simulink model "HANcoder_E407_TTA_Controller_v2"  (R2018b)
settings: Solver=FixedStepDiscrete  StartTime=0.0  StopTime=1  FixedStep=0.01  RelTol=1e-3
PreLoadFcn:
  | librarySetup
  | eval([bdroot,'_startup']) %Calling [modelName]_startup.m
values from neighbouring files (symbols this model uses):
  basic_cycle_duration_bc0 = TM_Reset_Board   + COMP_duration    (= 212)    [HANcoder_E407_TTA_Controller_v3_startup.m]
  basic_cycle_duration_bc1 = TM_Reset_Var_bc1 + COMP_duration    (= 288)    [HANcoder_E407_TTA_Controller_v3_startup.m]
  comm_delay_estimation1 = round(comm_delay_measured1*hardware_granularity/frequency_IRQ)    [HANcoder_E407_TTA_Controller_v3_startup.m]
  comm_delay_estimation2 = round(comm_delay_measured2*hardware_granularity/frequency_IRQ)    [HANcoder_E407_TTA_Controller_v3_startup.m]
  COMM_Period = 40    [HANcoder_E407_TTA_Controller_v3_startup.m]
  COMM_Phase1 = Simulink.Parameter    [HANcoder_E407_TTA_Controller_v3_startup.m]
  COMM_Phase2 = Simulink.Parameter    [HANcoder_E407_TTA_Controller_v3_startup.m]
  COMP_duration = 4    [HANcoder_E407_TTA_Controller_v3_startup.m]
  Controller1_Board = 1    [HANcoder_E407_TTA_Controller_v3_startup.m]
  Controller2_Board = 2    [HANcoder_E407_TTA_Controller_v3_startup.m]
  Controller3_Board = 3    [HANcoder_E407_TTA_Controller_v3_startup.m]
  delta_max = 1    [HANcoder_E407_TTA_Controller_v3_startup.m]
  delta_min = -1    [HANcoder_E407_TTA_Controller_v3_startup.m]
  delta_precision = 6    [HANcoder_E407_TTA_Controller_v3_startup.m]
  e_width = 0.1    [HANcoder_E407_TTA_Controller_v3_startup.m]
  frequency_IRQ = 100    [HANcoder_E407_TTA_Controller_v3_startup.m]
  HANtuneOverride = Simulink.Parameter    [HANcoder_E407_TTA_Controller_v3_startup.m]
  hardware_granularity = 1000000    [HANcoder_E407_TTA_Controller_v3_startup.m]
  I_a = 2.25    [HANcoder_E407_TTA_Controller_v3_startup.m]
  I_f = 2.25    [HANcoder_E407_TTA_Controller_v3_startup.m]
  idle_time_init = basic_cycle_duration_bc0 + basic_cycle_duration_bc1    (= 500)    [HANcoder_E407_TTA_Controller_v3_startup.m]
  Input_Gen_Board = 4    [HANcoder_E407_TTA_Controller_v3_startup.m]
  LA_Clock_Gr = 1    [HANcoder_E407_TTA_Controller_v3_startup.m]
  LA_COMM_Err = 1    [HANcoder_E407_TTA_Controller_v3_startup.m]
  LA_MEX_Flag = 1    [HANcoder_E407_TTA_Controller_v3_startup.m]
  LA_Task_Act = 1    [HANcoder_E407_TTA_Controller_v3_startup.m]
  m_v = 100.0    (= 100)    [HANcoder_E407_TTA_Controller_v3_startup.m]
  Master_Role = 1    [HANcoder_E407_TTA_Controller_v3_startup.m]
  matrix_cycle_duration = basic_cycle_duration_bc0 + basic_cycle_duration_bc1    (= 500)    [HANcoder_E407_TTA_Controller_v3_startup.m]
  matrix_rows = 2    [HANcoder_E407_TTA_Controller_v3_startup.m]
  max_num_msgs_CAN1 = 2^Tx_bit_number-1    (= 7)    [HANcoder_E407_TTA_Controller_v3_startup.m]
  max_num_msgs_CAN2 = max_num_msgs_CAN1    (= 7)    [HANcoder_E407_TTA_Controller_v3_startup.m]
  OutControl1_ID = 23    [HANcoder_E407_TTA_Controller_v3_startup.m]
  OutControl2_ID = 24    [HANcoder_E407_TTA_Controller_v3_startup.m]
  OutEmulator_ID = 25    [HANcoder_E407_TTA_Controller_v3_startup.m]
  R_al = 0.10    (= 0.1)    [HANcoder_E407_TTA_Controller_v3_startup.m]
  R_ar = 0.10    (= 0.1)    [HANcoder_E407_TTA_Controller_v3_startup.m]
  R_fl = 0.10    (= 0.1)    [HANcoder_E407_TTA_Controller_v3_startup.m]
  R_fr = 0.10    (= 0.1)    [HANcoder_E407_TTA_Controller_v3_startup.m]
  SensorValues_ID = 22    [HANcoder_E407_TTA_Controller_v3_startup.m]
  SetValues_ID = 21    [HANcoder_E407_TTA_Controller_v3_startup.m]
  Slave_Role = 2    [HANcoder_E407_TTA_Controller_v3_startup.m]
  speed_k_d = Simulink.Parameter    [HANcoder_E407_TTA_Controller_v3_startup.m]
  speed_k_i = Simulink.Parameter    [HANcoder_E407_TTA_Controller_v3_startup.m]
  speed_k_p = Simulink.Parameter    [HANcoder_E407_TTA_Controller_v3_startup.m]
  speed_max = 10    [HANcoder_E407_TTA_Controller_v3_startup.m]
  speed_min = -10    [HANcoder_E407_TTA_Controller_v3_startup.m]
  speed_precision = 3    [HANcoder_E407_TTA_Controller_v3_startup.m]
  Sync_ID = 1    [HANcoder_E407_TTA_Controller_v3_startup.m]
  tau_max = 5    [HANcoder_E407_TTA_Controller_v3_startup.m]
  tau_min = -5    [HANcoder_E407_TTA_Controller_v3_startup.m]
  tau_range = abs(tau_max) + abs(tau_min)    [HANcoder_E407_TTA_Controller_v3_startup.m]
  theta_max = (speed_max/R_fr)*matrix_cycle_duration*frequency_IRQ/hardware_granularity    (= 5)    [HANcoder_E407_TTA_Controller_v3_startup.m]
  theta_min = (-1)*theta_max    (= -5)    [HANcoder_E407_TTA_Controller_v3_startup.m]
  theta_precision = 7-(fix(log2(theta_max))+1)    [HANcoder_E407_TTA_Controller_v3_startup.m]
  Tl_a = 0.6    [HANcoder_E407_TTA_Controller_v3_startup.m]
  Tl_f = 0.6    [HANcoder_E407_TTA_Controller_v3_startup.m]
  TM_Check_Output_Control1 = TM_COMM_Output_Control1 + COMM_duration    (= 188)    [HANcoder_E407_TTA_Controller_v3_startup.m]
  TM_Check_Output_Control2 = TM_COMM_Output_Control2 + COMM_duration    (= 232)    [HANcoder_E407_TTA_Controller_v3_startup.m]
  TM_Check_Output_Emulator = TM_COMM_Output_Emulator + COMM_duration    (= 280)    [HANcoder_E407_TTA_Controller_v3_startup.m]
  TM_Check_Sensor_Values = TM_COMM_Sensor_Values + COMM_duration    (= 132)    [HANcoder_E407_TTA_Controller_v3_startup.m]
  TM_Check_Set_Values = TM_COMM_Set_Values + COMM_duration    (= 88)    [HANcoder_E407_TTA_Controller_v3_startup.m]
  TM_Check_Sync = TM_COMM_Sync   + COMM_duration    (= 40)    [HANcoder_E407_TTA_Controller_v3_startup.m]
  TM_Check_TOuts = TM_Count_Vote3 + COMP_duration    (= 196)    [HANcoder_E407_TTA_Controller_v3_startup.m]
  TM_Check_Vote1 = TM_COMM_Vote1  + COMM_duration    (= 92)    [HANcoder_E407_TTA_Controller_v3_startup.m]
  TM_Check_Vote2 = TM_COMM_Vote2  + COMM_duration    (= 140)    [HANcoder_E407_TTA_Controller_v3_startup.m]
  TM_Check_Vote3 = TM_COMM_Vote3  + COMM_duration    (= 188)    [HANcoder_E407_TTA_Controller_v3_startup.m]
  TM_COMM_Output_Control1 = TM_Velocity + COMP_duration    (= 148)    [HANcoder_E407_TTA_Controller_v3_startup.m]
  TM_COMM_Output_Control2 = TM_Check_Output_Control1 + COMP_duration    (= 192)    [HANcoder_E407_TTA_Controller_v3_startup.m]
  TM_COMM_Output_Emulator = TM_TMR + COMP_duration    (= 240)    [HANcoder_E407_TTA_Controller_v3_startup.m]
  TM_COMM_Sensor_Values = TM_Check_Set_Values + COMP_duration    (= 92)    [HANcoder_E407_TTA_Controller_v3_startup.m]
  TM_COMM_Set_Values = TM_Update_LT + COMP_duration    (= 48)    [HANcoder_E407_TTA_Controller_v3_startup.m]
  TM_COMM_Sync = basic_cycle_start    (= 0)    [HANcoder_E407_TTA_Controller_v3_startup.m]
  TM_COMM_Vote1 = TM_Vote_Dec    + COMP_duration    (= 52)    [HANcoder_E407_TTA_Controller_v3_startup.m]
  TM_COMM_Vote2 = TM_Count_Vote1 + COMP_duration    (= 100)    [HANcoder_E407_TTA_Controller_v3_startup.m]
  TM_COMM_Vote3 = TM_Count_Vote2 + COMP_duration    (= 148)    [HANcoder_E407_TTA_Controller_v3_startup.m]
  TM_Count_Vote1 = TM_Check_Vote1 + COMP_duration    (= 96)    [HANcoder_E407_TTA_Controller_v3_startup.m]
  TM_Count_Vote2 = TM_Check_Vote2 + COMP_duration    (= 144)    [HANcoder_E407_TTA_Controller_v3_startup.m]
  TM_Count_Vote3 = TM_Check_Vote3 + COMP_duration    (= 192)    [HANcoder_E407_TTA_Controller_v3_startup.m]
  TM_Data_bc0 = TM_COMM_Sync    (= 0)    [HANcoder_E407_TTA_Controller_v3_startup.m]
  TM_Data_bc1 = TM_Data_bc0(1:4)    [HANcoder_E407_TTA_Controller_v3_startup.m]
  TM_New_Master = TM_Check_TOuts + COMP_duration    (= 200)    [HANcoder_E407_TTA_Controller_v3_startup.m]
  TM_Reset_Board = TM_Reset_Var   + COMP_duration    (= 208)    [HANcoder_E407_TTA_Controller_v3_startup.m]
  TM_Reset_Var = TM_New_Master  + COMP_duration    (= 204)    [HANcoder_E407_TTA_Controller_v3_startup.m]
  TM_Reset_Var_bc1 = TM_Check_Output_Emulator + COMP_duration    (= 284)    [HANcoder_E407_TTA_Controller_v3_startup.m]
  TM_Steer = TM_Check_Sensor_Values + COMP_duration    (= 136)    [HANcoder_E407_TTA_Controller_v3_startup.m]
  TM_TMR = TM_Check_Output_Control2 + COMP_duration    (= 236)    [HANcoder_E407_TTA_Controller_v3_startup.m]
  TM_Torque = TM_Steer + COMP_duration    (= 140)    [HANcoder_E407_TTA_Controller_v3_startup.m]
  TM_Type_bc0 = COMM    (= 0)    [HANcoder_E407_TTA_Controller_v3_startup.m]
  TM_Type_bc1 = TM_Type_bc0(1:4)    [HANcoder_E407_TTA_Controller_v3_startup.m]
  TM_Update_LT = TM_Check_Sync  + COMP_duration    (= 44)    [HANcoder_E407_TTA_Controller_v3_startup.m]
  TM_Velocity = TM_Torque + COMP_duration    (= 144)    [HANcoder_E407_TTA_Controller_v3_startup.m]
  TM_Vote_Dec = TM_Update_LT   + COMP_duration    (= 48)    [HANcoder_E407_TTA_Controller_v3_startup.m]
  torque_a_k_d = Simulink.Parameter    [HANcoder_E407_TTA_Controller_v3_startup.m]
  torque_a_k_i = Simulink.Parameter    [HANcoder_E407_TTA_Controller_v3_startup.m]
  torque_a_k_p = Simulink.Parameter    [HANcoder_E407_TTA_Controller_v3_startup.m]
  torque_f_k_d = Simulink.Parameter    [HANcoder_E407_TTA_Controller_v3_startup.m]
  torque_f_k_i = Simulink.Parameter    [HANcoder_E407_TTA_Controller_v3_startup.m]
  torque_f_k_p = Simulink.Parameter    [HANcoder_E407_TTA_Controller_v3_startup.m]
  torque_precision = 4    [HANcoder_E407_TTA_Controller_v3_startup.m]
  Vehicle_Em_Board = 5    [HANcoder_E407_TTA_Controller_v3_startup.m]
  Vote1_ID = 11    [HANcoder_E407_TTA_Controller_v3_startup.m]
  Vote2_ID = 12    [HANcoder_E407_TTA_Controller_v3_startup.m]
  Vote3_ID = 13    [HANcoder_E407_TTA_Controller_v3_startup.m]
undefined symbols (not defined in the file or in its folder): A0, A1, A2, A3, A4, CON2
libraries: hdlsllib x235, HANcoder_STM32_Target x25, simulink x3, simulink_extras x1
(part 5 of 22)

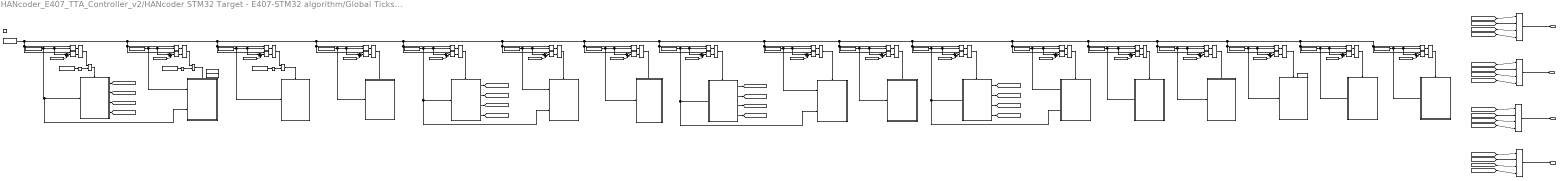
== system HANcoder_E407_TTA_Controller_v2/HANcoder STM32 Target - E407-STM32 algorithm/Global Ticks Increment/CAN Management/Matrix Cycle Manager/Subsystem/controller basic cycle 0 ==
  note: Output Send_Message
      | Send: 1
      | Do not send: 0
  note: Send message condition
      | Sync Msg: Master and TM0
      | Vote Msg: Node# and TM#
  note: Receive message condition
      | Sync Msg: Not Master and TM0
      | Vote Msg: Not # Node at TM#
  note: Receive message condition
      | Sync Msg: Not Master and TM0
      | Vote Msg: Not # Node at TM#
  note: Output Receive_Message
      | Receive: 1
      | Do not receive: 0
  note: Output Send_Message
      | Send: 1
      | Do not send: 0
  note: Output Receive_Message
      | Receive: 1
      | Do not receive: 0
  note: Send message condition
      | Sync Msg: Master and TM0
      | Vote Msg: Node# and TM#
  note: COMM - TW check
  note: COMP - TW check
  note: COMP - TW check
  note: COMP - TW check
  note: COMM - TW check
  note: COMP - TW check
  note: COMP - TW check
  note: COMM - TW check
  note: COMP - TW check
  note: COMP - TW check
  note: COMM - TW check
  note: COMP - TW check
  note: COMP - TW check
  note: COMP - TW check
  note: COMP - TW check
  note: COMP - TW check
  note: COMP - TW check
  note: Local Time still not updated
  note: Local Time still not updated
  note: Local Time still not updated
  Enable : EnablePort  PropagateVarSize=During execution
  AND{,1..19} (20 alike) : Logic  IconShape=distinctive  AllPortsSameDT=off  OutDataTypeStr=boolean
  COMM Task - Sync bc 0 : Subsystem
  COMM Task - Vote1 : Subsystem
  COMM Task - Vote2 : Subsystem
  COMM Task - Vote3 : Subsystem
  COMP Task - Check Timeouts : Subsystem
  COMP Task - New Master : Subsystem
  COMP Task - Reset Board : Subsystem
  COMP Task - Reset Variables BC0 : Subsystem
  COMP Task - Sync bc0 check : Subsystem
  COMP Task - Update LT : Subsystem
  COMP Task - Vote Decision : Subsystem
  COMP Task - Vote1 Count : Subsystem
  COMP Task - Vote1 check : Subsystem
  COMP Task - Vote2 Count : Subsystem
  COMP Task - Vote2 check : Subsystem
  COMP Task - Vote3 Count : Subsystem
  COMP Task - Vote3 check : Subsystem
  Constant : Constant  Value=TM_COMM_Sync
  Constant{1,4,10,29} (4 alike) : Constant  Value=COMM_Period
  Constant{5,7,11,13,15..16,18,20,22,24,26,30,32} (13 alike) : Constant  Value=COMP_duration
  Constant12 : Constant  Value=TM_Check_TOuts
  Constant14 : Constant  Value=TM_New_Master
  Constant17 : Constant  Value=TM_Update_LT
  Constant19 : Constant  Value=TM_Vote_Dec
  Constant2 : Constant  Value=TM_Check_Sync
  Constant21 : Constant  Value=TM_Count_Vote1
  Constant23 : Constant  Value=TM_Check_Vote3
  Constant25 : Constant  Value=TM_Reset_Var
  Constant27 : Constant  Value=TM_Count_Vote2
  Constant28 : Constant  Value=TM_COMM_Vote2
  Constant3 : Constant  Value=TM_COMM_Vote1
  Constant31 : Constant  Value=TM_Reset_Board
  Constant33 : Constant  Value=TM_Check_Vote2
  Constant6 : Constant  Value=TM_Check_Vote1
  Constant8 : Constant  Value=TM_Count_Vote3
  Constant9 : Constant  Value=TM_COMM_Vote3
  Data Store Memory11 : DataStoreMemory  DataStoreName=Msg_Rx  ReadBeforeWriteMsg=warning  WriteAfterWriteMsg=warning  WriteAfterReadMsg=warning  ShowAdditionalParam=off  OutDataTypeStr=Bus: msg_buffer_type
  Data Store Memory7 : DataStoreMemory  DataStoreName=Reset_Board  ReadBeforeWriteMsg=warning  WriteAfterWriteMsg=warning  WriteAfterReadMsg=warning  ShowAdditionalParam=off  OutDataTypeStr=boolean
  Data Store Memory8 : DataStoreMemory  DataStoreName=new_msg_Rx  ReadBeforeWriteMsg=warning  WriteAfterWriteMsg=warning  WriteAfterReadMsg=warning  ShowAdditionalParam=off
  Data Store Read11 : DataStoreRead  DataStoreName=BC0_Sync_processed
  Data Store Read6 : DataStoreRead  DataStoreName=BC0_Sync_processed
  Data Store Read7 : DataStoreRead  DataStoreName=BC0_Sync_processed
  Data Store Read8 : DataStoreRead  DataStoreName=Local_Ticks
  GreaterThan{,2,4,6,8,10,12,14,16,18,20,22,24,26,28,30,32} (17 alike) : RelationalOperator  OutDataTypeStr=boolean  RndMeth=Simplest
  GreaterThan{1,3,5,7,9,11,13,15,17,19,21,23,25,27,29,31,33} (17 alike) : RelationalOperator  Operator=<  OutDataTypeStr=boolean  RndMeth=Simplest
  NOT1 : Logic  Operator=NOT  IconShape=distinctive  AllPortsSameDT=off  OutDataTypeStr=boolean
  NOT2 : Logic  Operator=NOT  IconShape=distinctive  AllPortsSameDT=off  OutDataTypeStr=boolean
  NOT3 : Logic  Operator=NOT  IconShape=distinctive  AllPortsSameDT=off  OutDataTypeStr=boolean
  OR{1..4} (4 alike) : Logic  Operator=OR  Inputs=4  IconShape=distinctive  AllPortsSameDT=off  OutDataTypeStr=boolean
  Sum{1..17} (17 alike) : Sum  Inputs=|++
  Send_Message_CAN1 : Outport  OutputWhenDisabled=reset  InitialOutput=0
  Send_Message_CAN2 : Outport  Port=2  OutputWhenDisabled=reset  InitialOutput=0
  Receive_Message_CAN1 : Outport  Port=3  OutputWhenDisabled=reset  InitialOutput=0
  Receive_Message_CAN2 : Outport  Port=4  OutputWhenDisabled=reset  InitialOutput=0
  wires:
  OR1/1 -> Send_Message_CAN1/1
  [receive_CAN2_Sync_bc0_TAG] -> OR3/1
  [receive_CAN2_Vote3_bc0_TAG] -> OR3/4
  [receive_CAN2_Vote1_bc0_TAG] -> OR3/2
  [receive_CAN2_Vote2_bc0_TAG] -> OR3/3
  OR3/1 -> Receive_Message_CAN2/1
  [receive_CAN1_Sync_bc0_TAG] -> OR2/1
  [receive_CAN1_Vote1_bc0_TAG] -> OR2/2
  [receive_CAN1_Vote2_bc0_TAG] -> OR2/3
  [receive_CAN1_Vote3_bc0_TAG] -> OR2/4
  OR2/1 -> Receive_Message_CAN1/1
  [send_CAN2_Sync_bc0_TAG] -> OR4/1
  [send_CAN2_Vote1_bc0_TAG] -> OR4/2
  [send_CAN2_Vote2_bc0_TAG] -> OR4/3
  [send_CAN2_Vote3_bc0_TAG] -> OR4/4
  [send_CAN1_Sync_bc0_TAG] -> OR1/1
  [send_CAN1_Vote1_bc0_TAG] -> OR1/2
  [send_CAN1_Vote2_bc0_TAG] -> OR1/3
  [send_CAN1_Vote3_bc0_TAG] -> OR1/4
  OR4/1 -> Send_Message_CAN2/1
  COMM Task - Sync bc 0/1(Send CAN1) -> [send_CAN1_Sync_bc0_TAG]
  COMM Task - Sync bc 0/2(Receive CAN1) -> [receive_CAN1_Sync_bc0_TAG]
  COMM Task - Sync bc 0/3(Send CAN2) -> [send_CAN2_Sync_bc0_TAG]
  COMM Task - Sync bc 0/4(Receive CAN2) -> [receive_CAN2_Sync_bc0_TAG]
  Constant1/1 -> Sum4/2
  Constant/1 -> COMP Task - Sync bc0 check/2(TM_COMM), COMM Task - Sync bc 0/1(Time Mark), Sum4/1, GreaterThan/2
  Sum4/1 -> GreaterThan1/2
  GreaterThan/1 -> AND/1
  GreaterThan1/1 -> AND/2
  AND/1 -> AND17/1
  GreaterThan3/1 -> AND1/2
  GreaterThan2/1 -> AND1/1
  Sum1/1 -> GreaterThan3/2
  Constant2/1 -> COMP Task - Sync bc0 check/1(Time_Mark), GreaterThan2/2, Sum1/1
  Constant15/1 -> Sum1/2
  Constant16/1 -> Sum2/2
  Constant17/1 -> COMP Task - Update LT/1(Time_Mark), Sum2/1, GreaterThan4/2
  Sum2/1 -> GreaterThan5/2
  GreaterThan4/1 -> AND2/1
  GreaterThan5/1 -> AND2/2
  AND3/1 -> COMP Task - Vote Decision/Enable
  GreaterThan7/1 -> AND3/2
  GreaterThan6/1 -> AND3/1
  Sum3/1 -> GreaterThan7/2
  Constant19/1 -> COMP Task - Vote Decision/1(Time Mark), GreaterThan6/2, Sum3/1
  Constant18/1 -> Sum3/2
  COMM Task - Vote1/1(Send CAN1) -> [send_CAN1_Vote1_bc0_TAG]
  COMM Task - Vote1/2(Receive CAN1) -> [receive_CAN1_Vote1_bc0_TAG]
  COMM Task - Vote1/3(Send CAN2) -> [send_CAN2_Vote1_bc0_TAG]
  COMM Task - Vote1/4(Receive CAN2) -> [receive_CAN2_Vote1_bc0_TAG]
  GreaterThan9/1 -> AND4/2
  GreaterThan8/1 -> AND4/1
  Sum5/1 -> GreaterThan9/2
  Constant4/1 -> Sum5/2
  AND4/1 -> COMM Task - Vote1/Enable
  Constant3/1 -> COMP Task - Vote1 check/2(TM_COMM), COMM Task - Vote1/1(Time Mark), Sum5/1, GreaterThan8/2
  GreaterThan11/1 -> AND5/2
  Sum6/1 -> GreaterThan11/2
  GreaterThan10/1 -> AND5/1
  Constant5/1 -> Sum6/2
  Constant6/1 -> COMP Task - Vote1 check/1(Time_Mark), GreaterThan10/2, Sum6/1
  AND5/1 -> COMP Task - Vote1 check/Enable
  AND6/1 -> COMP Task - Vote1 Count/Enable
  Constant21/1 -> COMP Task - Vote1 Count/1(Time Mark), Sum7/1, GreaterThan12/2
  Constant20/1 -> Sum7/2
  GreaterThan12/1 -> AND6/1
  Sum7/1 -> GreaterThan13/2
  GreaterThan13/1 -> AND6/2
  GreaterThan17/1 -> AND9/2
  Sum10/1 -> GreaterThan17/2
  GreaterThan16/1 -> AND9/1
  Constant26/1 -> Sum10/2
  Constant27/1 -> COMP Task - Vote2 Count/1(Time Mark), GreaterThan16/2, Sum10/1
  AND9/1 -> COMP Task - Vote2 Count/Enable
  Constant33/1 -> COMP Task - Vote2 check/1(Time_Mark), Sum9/1, GreaterThan14/2
  Constant32/1 -> Sum9/2
  GreaterThan14/1 -> AND8/1
  Sum9/1 -> GreaterThan15/2
  GreaterThan15/1 -> AND8/2
  Constant28/1 -> COMP Task - Vote2 check/2(TM_COMM), COMM Task - Vote2/1(Time Mark), GreaterThan18/2, Sum8/1
  AND7/1 -> COMM Task - Vote2/Enable
  Constant29/1 -> Sum8/2
  Sum8/1 -> GreaterThan19/2
  GreaterThan18/1 -> AND7/1
  GreaterThan19/1 -> AND7/2
  COMM Task - Vote2/1(Send CAN1) -> [send_CAN1_Vote2_bc0_TAG]
  COMM Task - Vote2/2(Receive CAN1) -> [receive_CAN1_Vote2_bc0_TAG]
  COMM Task - Vote2/3(Send CAN2) -> [send_CAN2_Vote2_bc0_TAG]
  AND8/1 -> COMP Task - Vote2 check/Enable
  GreaterThan25/1 -> AND10/2
  GreaterThan24/1 -> AND10/1
  Sum12/1 -> GreaterThan25/2
  Constant10/1 -> Sum12/2
  Constant9/1 -> COMP Task - Vote3 check/2(TM_COMM), COMM Task - Vote3/1(Time Mark), Sum12/1, GreaterThan24/2
  GreaterThan21/1 -> AND11/2
  Sum13/1 -> GreaterThan21/2
  GreaterThan20/1 -> AND11/1
  Constant22/1 -> Sum13/2
  Constant23/1 -> COMP Task - Vote3 check/1(Time_Mark), GreaterThan20/2, Sum13/1
  AND12/1 -> COMP Task - Vote3 Count/Enable
  Constant8/1 -> COMP Task - Vote3 Count/1(Time Mark), Sum11/1, GreaterThan22/2
  Constant7/1 -> Sum11/2
  GreaterThan22/1 -> AND12/1
  Sum11/1 -> GreaterThan23/2
  GreaterThan23/1 -> AND12/2
  COMM Task - Vote3/1(Send CAN1) -> [send_CAN1_Vote3_bc0_TAG]
  COMM Task - Vote3/2(Receive CAN1) -> [receive_CAN1_Vote3_bc0_TAG]
  COMM Task - Vote3/3(Send CAN2) -> [send_CAN2_Vote3_bc0_TAG]
  COMM Task - Vote3/4(Receive CAN2) -> [receive_CAN2_Vote3_bc0_TAG]
  AND10/1 -> COMM Task - Vote3/Enable
  AND11/1 -> COMP Task - Vote3 check/Enable
  GreaterThan27/1 -> AND13/2
  Sum14/1 -> GreaterThan27/2
  GreaterThan26/1 -> AND13/1
  Constant11/1 -> Sum14/2
  Constant12/1 -> COMP Task - Check Timeouts/1(Time_Mark), GreaterThan26/2, Sum14/1
  AND13/1 -> COMP Task - Check Timeouts/Enable
  AND14/1 -> COMP Task - New Master/Enable
  Constant14/1 -> COMP Task - New Master/1(Time_Mark), Sum15/1, GreaterThan28/2
  Constant13/1 -> Sum15/2
  GreaterThan28/1 -> AND14/1
  Sum15/1 -> GreaterThan29/2
  GreaterThan29/1 -> AND14/2
  GreaterThan31/1 -> AND15/2
  Sum16/1 -> GreaterThan31/2
  GreaterThan30/1 -> AND15/1
  Constant24/1 -> Sum16/2
  Constant25/1 -> COMP Task - Reset Variables BC0/1(Time_Mark), GreaterThan30/2, Sum16/1
  AND15/1 -> COMP Task - Reset Variables BC0/Enable
  Data Store Read8/1 -> GreaterThan21/1, GreaterThan20/1, GreaterThan22/1, GreaterThan23/1, GreaterThan32/1, GreaterThan33/1, GreaterThan31/1, GreaterThan30/1, GreaterThan28/1, GreaterThan29/1, GreaterThan27/1, GreaterThan26/1, GreaterThan25/1, GreaterThan24/1, GreaterThan17/1, GreaterThan16/1, GreaterThan14/1, GreaterThan15/1, GreaterThan18/1, GreaterThan19/1, GreaterThan12/1, GreaterThan13/1, GreaterThan11/1, GreaterThan10/1, GreaterThan9/1, GreaterThan8/1, GreaterThan6/1, GreaterThan7/1, GreaterThan4/1, GreaterThan5/1, GreaterThan2/1, GreaterThan3/1, GreaterThan/1, GreaterThan1/1
  AND16/1 -> COMP Task - Reset Board/Enable
  Constant31/1 -> COMP Task - Reset Board/1(Time_Mark), Sum17/1, GreaterThan32/2
  Constant30/1 -> Sum17/2
  GreaterThan32/1 -> AND16/1
  Sum17/1 -> GreaterThan33/2
  GreaterThan33/1 -> AND16/2
  Data Store Read11/1 -> NOT2/1
  NOT2/1 -> AND17/2
  AND17/1 -> COMM Task - Sync bc 0/Enable
  Data Store Read6/1 -> NOT1/1
  NOT1/1 -> AND18/2
  AND1/1 -> AND18/1
  AND18/1 -> COMP Task - Sync bc0 check/Enable
  Data Store Read7/1 -> NOT3/1
  NOT3/1 -> AND19/2
  AND2/1 -> AND19/1
  AND19/1 -> COMP Task - Update LT/Enable
  COMM Task - Vote2/4(Receive CAN2) -> [receive_CAN2_Vote2_bc0_TAG]

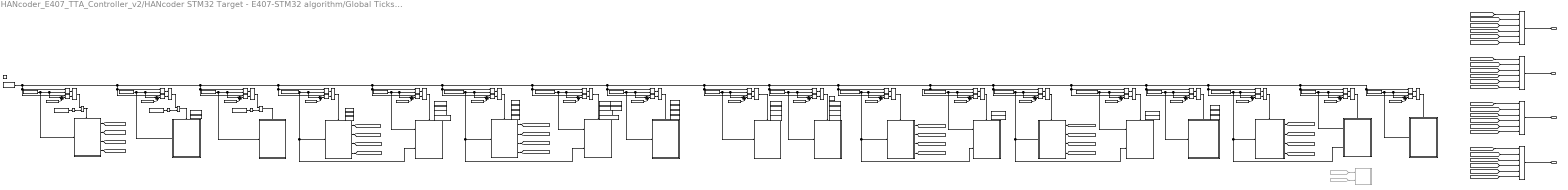
== system HANcoder_E407_TTA_Controller_v2/HANcoder STM32 Target - E407-STM32 algorithm/Global Ticks Increment/CAN Management/Matrix Cycle Manager/Subsystem/controller basic cycle 1 ==
  note: Receive message condition
      | Sync Msg: Not Master and TM0
      | Vote Msg: Not # Node at TM#
  note: Send message condition
      | Sync Msg: Master and TM0
      | Vote Msg: Node# and TM#
  note: Output Send_Message
      | Send: 1
      | Do not send: 0
  note: Output Receive_Message
      | Receive: 1
      | Do not receive: 0
  note: Output Receive_Message
      | Receive: 1
      | Do not receive: 0
  note: Output Send_Message
      | Send: 1
      | Do not send: 0
  note: Send message condition
      | Sync Msg: Master and TM0
      | Vote Msg: Node# and TM#
  note: Receive message condition
      | Sync Msg: Not Master and TM0
      | Vote Msg: Not # Node at TM#
  note: COMM - TW check
  note: COMP - TW check
  note: COMM - TW check
  note: COMP - TW check
  note: COMP - TW check
  note: COMP - TW check
  note: COMP - TW check
  note: COMM - TW check
  note: COMP - TW check
  note: COMP - TW check
  note: COMP - TW check
  note: Local Time still not updated
  note: COMP - TW check
  note: COMP - TW check
  note: Local Time still not updated
  note: COMP - TW check
  note: COMP - TW check
  note: COMM - TW check
  note: Local Time still not updated
  note: COMM - TW check
  note: COMP - TW check
  Enable : EnablePort
  AND{,1..20} (21 alike) : Logic  IconShape=distinctive  AllPortsSameDT=off  OutDataTypeStr=boolean
  COMM Task - Output Control1 : Subsystem
  COMM Task - Output Control2 : Subsystem
  COMM Task - Output Emulator : Subsystem
  COMM Task - Sensor_Values : Subsystem
  COMM Task - Set_Values : Subsystem
  COMM Task - Sync bc 1 : Subsystem
  COMP Task - Calculate Speed : Subsystem
  COMP Task - Calculate Steer : Subsystem
  COMP Task - Calculate Torque : Subsystem
  COMP Task - Estimate Vehicle States : Subsystem  Commented=on
  COMP Task - Reset Variables BC1 : Subsystem
  COMP Task - Rx_Output_Control1_Check : Subsystem
  COMP Task - Rx_Output_Control2_Check : Subsystem
  COMP Task - Rx_Output_Emulator_Check : Subsystem
  COMP Task - Rx_Sensor_Values_Check : Subsystem
  COMP Task - Rx_Set_Values_Check : Subsystem
  COMP Task - Sync bc1 check : Subsystem
  COMP Task - TMR : Subsystem
  COMP Task - Update LT : Subsystem
  Constant : Constant  Value=TM_COMM_Sync
  Constant{1,10,18,24,34,36} (6 alike) : Constant  Value=COMM_Period
  Constant{2..3,8..9,11,13,15,20,22,26,29..30} (12 alike) : Constant  Value=COMP_duration
  Constant12 : Constant  Value=TM_Check_Output_Control2
  Constant14 : Constant  Value=TM_TMR
  Constant16 : Constant  Value=TM_Reset_Var_bc1
  Constant21 : Constant  Value=TM_Check_Sensor_Values
  Constant23 : Constant  Value=TM_Check_Output_Control1
  Constant25 : Constant  Value=TM_COMM_Output_Emulator
  Constant27 : Constant  Value=TM_Velocity
  Constant28 : Constant  Value=TM_Steer
  Constant31 : Constant  Value=TM_Reset_Board
  Constant33 : Constant  Value=TM_Torque
  Constant35 : Constant  Value=TM_COMM_Sensor_Values
  Constant37 : Constant  Value=TM_COMM_Output_Control2
  Constant38 : Constant  Value=TM_COMM_Output_Control1
  Constant4 : Constant  Value=TM_Update_LT
  Constant5 : Constant  Value=TM_COMM_Set_Values
  Constant6 : Constant  Value=TM_Check_Sync
  Constant7 : Constant  Value=TM_Check_Set_Values
  Data Store Memory10 : DataStoreMemory  DataStoreName=v_set_stored  ReadBeforeWriteMsg=warning  WriteAfterWriteMsg=warning  WriteAfterReadMsg=warning  ShowAdditionalParam=off
  Data Store Memory11 : DataStoreMemory  DataStoreName=Msg_Rx  ReadBeforeWriteMsg=warning  WriteAfterWriteMsg=warning  WriteAfterReadMsg=warning  ShowAdditionalParam=off  OutDataTypeStr=Bus: msg_buffer_type
  Data Store Memory13 : DataStoreMemory  DataStoreName=theta_ar_stored  ReadBeforeWriteMsg=warning  WriteAfterWriteMsg=warning  WriteAfterReadMsg=warning  ShowAdditionalParam=off
  Data Store Memory14 : DataStoreMemory  DataStoreName=theta_al_stored  ReadBeforeWriteMsg=warning  WriteAfterWriteMsg=warning  WriteAfterReadMsg=warning  ShowAdditionalParam=off
  Data Store Memory18 : DataStoreMemory  DataStoreName=rx_data_incr_time  ReadBeforeWriteMsg=warning  WriteAfterWriteMsg=warning  WriteAfterReadMsg=warning  InitialValue=1  ShowAdditionalParam=off
  Data Store Memory19 : DataStoreMemory  DataStoreName=output_control1_rx  ReadBeforeWriteMsg=warning  WriteAfterWriteMsg=warning  WriteAfterReadMsg=warning  ShowAdditionalParam=off
  Data Store Memory20 : DataStoreMemory  DataStoreName=delta_f_set_stored  ReadBeforeWriteMsg=warning  WriteAfterWriteMsg=warning  WriteAfterReadMsg=warning  ShowAdditionalParam=off
  Data Store Memory21 : DataStoreMemory  DataStoreName=torque_fr_out  ReadBeforeWriteMsg=warning  WriteAfterWriteMsg=warning  WriteAfterReadMsg=warning  ShowAdditionalParam=off
  Data Store Memory22 : DataStoreMemory  DataStoreName=torque_fl_out  ReadBeforeWriteMsg=warning  WriteAfterWriteMsg=warning  WriteAfterReadMsg=warning  ShowAdditionalParam=off
  Data Store Memory23 : DataStoreMemory  DataStoreName=v_set  ReadBeforeWriteMsg=warning  WriteAfterWriteMsg=warning  WriteAfterReadMsg=warning  ShowAdditionalParam=off
  Data Store Memory24 : DataStoreMemory  DataStoreName=delta_f_set  ReadBeforeWriteMsg=warning  WriteAfterWriteMsg=warning  WriteAfterReadMsg=warning  ShowAdditionalParam=off
  Data Store Memory25 : DataStoreMemory  DataStoreName=torque_ar_out  ReadBeforeWriteMsg=warning  WriteAfterWriteMsg=warning  WriteAfterReadMsg=warning  ShowAdditionalParam=off
  Data Store Memory26 : DataStoreMemory  DataStoreName=torque_al_out  ReadBeforeWriteMsg=warning  WriteAfterWriteMsg=warning  WriteAfterReadMsg=warning  ShowAdditionalParam=off
  Data Store Memory27 : DataStoreMemory  DataStoreName=delta_a_set  ReadBeforeWriteMsg=warning  WriteAfterWriteMsg=warning  WriteAfterReadMsg=warning  ShowAdditionalParam=off
  Data Store Memory28 : DataStoreMemory  DataStoreName=Error_SetValues_NotRX  ReadBeforeWriteMsg=warning  WriteAfterWriteMsg=warning  WriteAfterReadMsg=warning  ShowAdditionalParam=off  OutDataTypeStr=boolean
  Data Store Memory30 : DataStoreMemory  DataStoreName=Error_SensorValues_NotRX  ReadBeforeWriteMsg=warning  WriteAfterWriteMsg=warning  WriteAfterReadMsg=warning  ShowAdditionalParam=off  OutDataTypeStr=boolean
  Data Store Memory31 : DataStoreMemory  DataStoreName=delta_a_set_stored  ReadBeforeWriteMsg=warning  WriteAfterWriteMsg=warning  WriteAfterReadMsg=warning  ShowAdditionalParam=off
  Data Store Memory33 : DataStoreMemory  DataStoreName=theta_fr  ReadBeforeWriteMsg=warning  WriteAfterWriteMsg=warning  WriteAfterReadMsg=warning  ShowAdditionalParam=off
  Data Store Memory34 : DataStoreMemory  DataStoreName=theta_dot_fr  ReadBeforeWriteMsg=warning  WriteAfterWriteMsg=warning  WriteAfterReadMsg=warning  ShowAdditionalParam=off
  Data Store Memory35 : DataStoreMemory  DataStoreName=theta_dot_ar  ReadBeforeWriteMsg=warning  WriteAfterWriteMsg=warning  WriteAfterReadMsg=warning  ShowAdditionalParam=off
  Data Store Memory36 : DataStoreMemory  DataStoreName=theta_dot_fl  ReadBeforeWriteMsg=warning  WriteAfterWriteMsg=warning  WriteAfterReadMsg=warning  ShowAdditionalParam=off
  Data Store Memory37 : DataStoreMemory  DataStoreName=theta_dot_al  ReadBeforeWriteMsg=warning  WriteAfterWriteMsg=warning  WriteAfterReadMsg=warning  ShowAdditionalParam=off
  Data Store Memory38 : DataStoreMemory  DataStoreName=v_est  ReadBeforeWriteMsg=warning  WriteAfterWriteMsg=warning  WriteAfterReadMsg=warning  ShowAdditionalParam=off
  Data Store Memory39 : DataStoreMemory  DataStoreName=torque_fr_set  ReadBeforeWriteMsg=warning  WriteAfterWriteMsg=warning  WriteAfterReadMsg=warning  ShowAdditionalParam=off
  Data Store Memory40 : DataStoreMemory  DataStoreName=torque_fl_set  ReadBeforeWriteMsg=warning  WriteAfterWriteMsg=warning  WriteAfterReadMsg=warning  ShowAdditionalParam=off
  Data Store Memory41 : DataStoreMemory  DataStoreName=torque_ar_set  ReadBeforeWriteMsg=warning  WriteAfterWriteMsg=warning  WriteAfterReadMsg=warning  ShowAdditionalParam=off
  Data Store Memory42 : DataStoreMemory  DataStoreName=torque_al_set  ReadBeforeWriteMsg=warning  WriteAfterWriteMsg=warning  WriteAfterReadMsg=warning  ShowAdditionalParam=off
  Data Store Memory43 : DataStoreMemory  DataStoreName=theta_fl  ReadBeforeWriteMsg=warning  WriteAfterWriteMsg=warning  WriteAfterReadMsg=warning  ShowAdditionalParam=off
  Data Store Memory44 : DataStoreMemory  DataStoreName=theta_ar  ReadBeforeWriteMsg=warning  WriteAfterWriteMsg=warning  WriteAfterReadMsg=warning  ShowAdditionalParam=off
  Data Store Memory46 : DataStoreMemory  DataStoreName=theta_al  ReadBeforeWriteMsg=warning  WriteAfterWriteMsg=warning  WriteAfterReadMsg=warning  ShowAdditionalParam=off
  Data Store Memory47 : DataStoreMemory  DataStoreName=output_control1_msg  ReadBeforeWriteMsg=warning  WriteAfterWriteMsg=warning  WriteAfterReadMsg=warning  ShowAdditionalParam=off  OutDataTypeStr=Bus: msg_buffer_type
  Data Store Memory48 : DataStoreMemory  DataStoreName=output_control2_rx  ReadBeforeWriteMsg=warning  WriteAfterWriteMsg=warning  WriteAfterReadMsg=warning  ShowAdditionalParam=off
  Data Store Memory49 : DataStoreMemory  DataStoreName=output_control2_msg  ReadBeforeWriteMsg=warning  WriteAfterWriteMsg=warning  WriteAfterReadMsg=warning  ShowAdditionalParam=off  OutDataTypeStr=Bus: msg_buffer_type
  Data Store Memory50 : DataStoreMemory  DataStoreName=error_log_1  ReadBeforeWriteMsg=warning  WriteAfterWriteMsg=warning  WriteAfterReadMsg=warning  ShowAdditionalParam=off  OutDataTypeStr=uint8
  Data Store Memory51 : DataStoreMemory  DataStoreName=theta_fr_stored  ReadBeforeWriteMsg=warning  WriteAfterWriteMsg=warning  WriteAfterReadMsg=warning  ShowAdditionalParam=off
  Data Store Memory52 : DataStoreMemory  DataStoreName=theta_fl_stored  ReadBeforeWriteMsg=warning  WriteAfterWriteMsg=warning  WriteAfterReadMsg=warning  ShowAdditionalParam=off
  Data Store Memory53 : DataStoreMemory  DataStoreName=error_log_2  ReadBeforeWriteMsg=warning  WriteAfterWriteMsg=warning  WriteAfterReadMsg=warning  ShowAdditionalParam=off  OutDataTypeStr=uint8
  Data Store Memory54 : DataStoreMemory  DataStoreName=error_log_3  ReadBeforeWriteMsg=warning  WriteAfterWriteMsg=warning  WriteAfterReadMsg=warning  ShowAdditionalParam=off  OutDataTypeStr=uint8
  Data Store Memory8 : DataStoreMemory  DataStoreName=new_msg_Rx  ReadBeforeWriteMsg=warning  WriteAfterWriteMsg=warning  WriteAfterReadMsg=warning  ShowAdditionalParam=off
  Data Store Read1 : DataStoreRead  DataStoreName=Local_Ticks
  Data Store Read11 : DataStoreRead  DataStoreName=BC1_Sync_processed
  Data Store Read6 : DataStoreRead  DataStoreName=BC1_Sync_processed
  Data Store Read7 : DataStoreRead  DataStoreName=BC1_Sync_processed
  From180 : From  Commented=on  GotoTag=basic_cycle_TAG
  From181 : From  Commented=on  GotoTag=local_ticks_TAG
  GreaterThan{,2,4,6,8,10,12,14,16,18,20,22,24,26,28,30,32,34} (18 alike) : RelationalOperator  OutDataTypeStr=boolean  RndMeth=Simplest
  GreaterThan{1,3,5,7,9,11,13,15,17,19,21,23,25,27,29,31,33,35} (18 alike) : RelationalOperator  Operator=<  OutDataTypeStr=boolean  RndMeth=Simplest
  NOT2 : Logic  Operator=NOT  IconShape=distinctive  AllPortsSameDT=off  OutDataTypeStr=boolean
  NOT4 : Logic  Operator=NOT  IconShape=distinctive  AllPortsSameDT=off  OutDataTypeStr=boolean
  NOT5 : Logic  Operator=NOT  IconShape=distinctive  AllPortsSameDT=off  OutDataTypeStr=boolean
  OR{1..4} (4 alike) : Logic  Operator=OR  Inputs=6  IconShape=distinctive  AllPortsSameDT=off  OutDataTypeStr=boolean
  Sum{1..18} (18 alike) : Sum  Inputs=|++
  Send_Message_CAN1 : Outport  OutputWhenDisabled=reset  InitialOutput=0
  Send_Message_CAN2 : Outport  Port=2  OutputWhenDisabled=reset  InitialOutput=0
  Receive_Message_CAN1 : Outport  Port=3  OutputWhenDisabled=reset  InitialOutput=0
  Receive_Message_CAN2 : Outport  Port=4  OutputWhenDisabled=reset  InitialOutput=0
  wires:
  COMM Task - Sensor_Values/3(Send CAN2) -> [send_CAN2_Sensor_Values_bc1_TAG]
  COMM Task - Sensor_Values/1(Send CAN1) -> [send_CAN1_Sensor_Values_bc1_TAG]
  COMM Task - Sensor_Values/2(Receive CAN1) -> [receive_CAN1_Sensor_Values_bc1_TAG]
  COMM Task - Sensor_Values/4(Receive CAN2) -> [receive_CAN2_Sensor_Values_bc1_TAG]
  From181/1 -> COMP Task - Estimate Vehicle States/2(local time)
  From180/1 -> COMP Task - Estimate Vehicle States/1(basic cycle)
  OR1/1 -> Send_Message_CAN1/1
  OR2/1 -> Receive_Message_CAN2/1
  OR4/1 -> Send_Message_CAN2/1
  OR3/1 -> Receive_Message_CAN1/1
  [send_CAN1_Sync_bc1_TAG] -> OR1/1
  [send_CAN1_Set_Values_bc1_TAG] -> OR1/2
  [send_CAN1_Sensor_Values_bc1_TAG] -> OR1/3
  [send_CAN1_Out_Control1_bc1_TAG] -> OR1/4
  [send_CAN1_Out_Control2_bc1_TAG] -> OR1/5
  [send_CAN1_Out_Emulator_bc1_TAG] -> OR1/6
  [send_CAN2_Sync_bc1_TAG] -> OR4/1
  [send_CAN2_Set_Values_bc1_TAG] -> OR4/2
  [send_CAN2_Sensor_Values_bc1_TAG] -> OR4/3
  [send_CAN2_Out_Control1_bc1_TAG] -> OR4/4
  [send_CAN2_Out_Control2_bc1_TAG] -> OR4/5
  [send_CAN2_Out_Emulator_bc1_TAG] -> OR4/6
  [receive_CAN1_Sync_bc1_TAG] -> OR3/1
  [receive_CAN1_Set_Values_bc1_TAG] -> OR3/2
  [receive_CAN1_Sensor_Values_bc1_TAG] -> OR3/3
  [receive_CAN1_Out_Control1_bc1_TAG] -> OR3/4
  [receive_CAN1_Out_Emulator_bc1_TAG] -> OR3/6
  [receive_CAN1_Out_Control2_bc1_TAG] -> OR3/5
  [receive_CAN2_Sync_bc1_TAG] -> OR2/1
  [receive_CAN2_Set_Values_bc1_TAG] -> OR2/2
  [receive_CAN2_Out_Control1_bc1_TAG] -> OR2/4
  [receive_CAN2_Sensor_Values_bc1_TAG] -> OR2/3
  [receive_CAN2_Out_Control2_bc1_TAG] -> OR2/5
  [receive_CAN2_Out_Emulator_bc1_TAG] -> OR2/6
  AND11/1 -> COMP Task - Rx_Output_Control1_Check/Enable
  AND12/1 -> COMM Task - Output Control2/Enable
  Constant1/1 -> Sum4/2
  COMM Task - Sync bc 1/1(Send CAN1) -> [send_CAN1_Sync_bc1_TAG]
  COMM Task - Sync bc 1/2(Receive CAN1) -> [receive_CAN1_Sync_bc1_TAG]
  COMM Task - Sync bc 1/4(Receive CAN2) -> [receive_CAN2_Sync_bc1_TAG]
  GreaterThan18/1 -> AND7/1
  AND19/1 -> COMP Task - Update LT/Enable
  AND4/1 -> COMP Task - Rx_Set_Values_Check/Enable
  Constant38/1 -> COMP Task - Rx_Output_Control1_Check/2(TM_COMM), COMM Task - Output Control1/1(Time Mark), Sum12/1, GreaterThan24/2
  GreaterThan29/1 -> AND14/2
  NOT2/1 -> AND18/2
  Constant14/1 -> COMP Task - TMR/1(Time_Mark), Sum15/1, GreaterThan28/2
  Sum15/1 -> GreaterThan29/2
  GreaterThan24/1 -> AND10/1
  GreaterThan16/1 -> AND9/1
  Constant9/1 -> Sum5/2
  GreaterThan22/1 -> AND12/1
  Sum14/1 -> GreaterThan27/2
  Data Store Read7/1 -> NOT5/1
  GreaterThan4/1 -> AND2/1
  Constant31/1 -> COMP Task - Rx_Output_Emulator_Check/1(Time_Mark), Sum17/1, GreaterThan32/2
  AND3/1 -> COMM Task - Set_Values/Enable
  GreaterThan28/1 -> AND14/1
  AND18/1 -> COMP Task - Sync bc1 check/Enable
  GreaterThan12/1 -> AND6/1
  AND1/1 -> AND18/1
  Sum17/1 -> GreaterThan33/2
  Constant30/1 -> Sum17/2
  GreaterThan20/1 -> AND11/1
  Data Store Read11/1 -> NOT4/1
  AND13/1 -> COMP Task - Rx_Output_Control2_Check/Enable
  AND17/1 -> COMM Task - Sync bc 1/Enable
  GreaterThan25/1 -> AND10/2
  GreaterThan33/1 -> AND16/2
  AND2/1 -> AND19/1
  GreaterThan32/1 -> AND16/1
  Data Store Read6/1 -> NOT2/1
  NOT4/1 -> AND17/2
  GreaterThan23/1 -> AND12/2
  AND15/1 -> COMM Task - Output Emulator/Enable
  AND14/1 -> COMP Task - TMR/Enable
  AND16/1 -> COMP Task - Rx_Output_Emulator_Check/Enable
  GreaterThan30/1 -> AND15/1
  Sum16/1 -> GreaterThan31/2
  Constant24/1 -> Sum16/2
  Constant25/1 -> COMP Task - Rx_Output_Emulator_Check/2(TM_COMM), COMM Task - Output Emulator/1(Time Mark), GreaterThan30/2, Sum16/1
  Constant27/1 -> COMP Task - Calculate Speed/1(Time_Mark), GreaterThan16/2, Sum10/1
  GreaterThan21/1 -> AND11/2
  GreaterThan1/1 -> AND/2
  Constant13/1 -> Sum15/2
  GreaterThan/1 -> AND/1
  Constant37/1 -> Sum11/1, GreaterThan22/2, COMP Task - Rx_Output_Control2_Check/2(TM_COMM), COMM Task - Output Control2/1(Time Mark)
  Constant20/1 -> Sum7/2
  Constant12/1 -> COMP Task - Rx_Output_Control2_Check/1(Time_Mark), GreaterThan26/2, Sum14/1
  GreaterThan10/1 -> AND5/1
  Constant/1 -> COMM Task - Sync bc 1/1(Time Mark), Sum4/1, GreaterThan/2
  GreaterThan26/1 -> AND13/1
  Constant11/1 -> Sum14/2
  AND7/1 -> COMP Task - Calculate Steer/Enable
  Constant23/1 -> COMP Task - Rx_Output_Control1_Check/1(Time_Mark), GreaterThan20/2, Sum13/1
  Constant5/1 -> COMM Task - Set_Values/1(Time Mark), COMP Task - Rx_Set_Values_Check/2(TM_COMM), GreaterThan6/2, Sum3/1
  Sum12/1 -> GreaterThan25/2
  Sum11/1 -> GreaterThan23/2
  Constant18/1 -> Sum3/2
  Constant22/1 -> Sum13/2
  GreaterThan19/1 -> AND7/2
  Sum8/1 -> GreaterThan19/2
  Constant10/1 -> Sum12/2
  Sum9/1 -> GreaterThan15/2
  Constant29/1 -> Sum8/2
  AND/1 -> AND17/1
  Constant28/1 -> COMP Task - Calculate Steer/1(Time_Mark), GreaterThan18/2, Sum8/1
  GreaterThan15/1 -> AND8/2
  Constant26/1 -> Sum10/2
  Sum10/1 -> GreaterThan17/2
  GreaterThan14/1 -> AND8/1
  Constant8/1 -> Sum9/2
  Sum7/1 -> GreaterThan13/2
  Constant36/1 -> Sum11/2
  Sum6/1 -> GreaterThan11/2
  Constant3/1 -> Sum2/2
  Constant35/1 -> COMP Task - Rx_Sensor_Values_Check/2(TM_COMM), COMM Task - Sensor_Values/1(Time Mark), GreaterThan10/2, Sum6/1
  Constant7/1 -> COMP Task - Rx_Set_Values_Check/1(Time_Mark), Sum5/1, GreaterThan8/2
  GreaterThan17/1 -> AND9/2
  AND10/1 -> COMM Task - Output Control1/Enable
  Sum3/1 -> GreaterThan7/2
  Constant4/1 -> COMP Task - Update LT/1(Time_Mark), Sum2/1, GreaterThan4/2
  Sum5/1 -> GreaterThan9/2
  Sum4/1 -> GreaterThan1/2
  AND5/1 -> COMM Task - Sensor_Values/Enable
  GreaterThan6/1 -> AND3/1
  GreaterThan8/1 -> AND4/1
  GreaterThan9/1 -> AND4/2
  GreaterThan31/1 -> AND15/2
  AND8/1 -> COMP Task - Calculate Torque/Enable
  GreaterThan13/1 -> AND6/2
  Sum13/1 -> GreaterThan21/2
  GreaterThan2/1 -> AND1/1
  GreaterThan3/1 -> AND1/2
  Constant2/1 -> Sum1/2
  GreaterThan7/1 -> AND3/2
  Constant6/1 -> COMP Task - Sync bc1 check/1(Time_Mark), GreaterThan2/2, Sum1/1
  AND6/1 -> COMP Task - Rx_Sensor_Values_Check/Enable
  GreaterThan11/1 -> AND5/2
  Sum1/1 -> GreaterThan3/2
  Constant34/1 -> Sum6/2
  AND9/1 -> COMP Task - Calculate Speed/Enable
  COMM Task - Sync bc 1/3(Send CAN2) -> [send_CAN2_Sync_bc1_TAG]
  Constant33/1 -> COMP Task - Calculate Torque/1(Time_Mark), Sum9/1, GreaterThan14/2
  GreaterThan27/1 -> AND13/2
  Constant21/1 -> COMP Task - Rx_Sensor_Values_Check/1(Time_Mark), Sum7/1, GreaterThan12/2
  NOT5/1 -> AND19/2
  Sum2/1 -> GreaterThan5/2
  GreaterThan5/1 -> AND2/2
  COMM Task - Set_Values/1(Send CAN1) -> [send_CAN1_Set_Values_bc1_TAG]
  COMM Task - Set_Values/2(Receive CAN1) -> [receive_CAN1_Set_Values_bc1_TAG]
  COMM Task - Set_Values/3(Send CAN2) -> [send_CAN2_Set_Values_bc1_TAG]
  COMM Task - Set_Values/4(Receive CAN2) -> [receive_CAN2_Set_Values_bc1_TAG]
  COMM Task - Output Control1/1(Send CAN1) -> [send_CAN1_Out_Control1_bc1_TAG]
  COMM Task - Output Control1/2(Receive CAN1) -> [receive_CAN1_Out_Control1_bc1_TAG]
  COMM Task - Output Control1/4(Receive CAN2) -> [receive_CAN2_Out_Control1_bc1_TAG]
  COMM Task - Output Control1/3(Send CAN2) -> [send_CAN2_Out_Control1_bc1_TAG]
  COMM Task - Output Control2/1(Send CAN1) -> [send_CAN1_Out_Control2_bc1_TAG]
  COMM Task - Output Control2/2(Receive CAN1) -> [receive_CAN1_Out_Control2_bc1_TAG]
  COMM Task - Output Control2/3(Send CAN2) -> [send_CAN2_Out_Control2_bc1_TAG]
  COMM Task - Output Control2/4(Receive CAN2) -> [receive_CAN2_Out_Control2_bc1_TAG]
  GreaterThan35/1 -> AND20/2
  Constant16/1 -> Sum18/1, GreaterThan34/2, COMP Task - Reset Variables BC1/1(Time_Mark)
  Constant15/1 -> Sum18/2
  Sum18/1 -> GreaterThan35/2
  GreaterThan34/1 -> AND20/1
  AND20/1 -> COMP Task - Reset Variables BC1/Enable
  Data Store Read1/1 -> GreaterThan34/1, GreaterThan35/1, GreaterThan32/1, GreaterThan33/1, GreaterThan30/1, GreaterThan31/1, GreaterThan28/1, GreaterThan29/1, GreaterThan26/1, GreaterThan27/1, GreaterThan23/1, GreaterThan22/1, GreaterThan21/1, GreaterThan20/1, GreaterThan24/1, GreaterThan25/1, GreaterThan16/1, GreaterThan17/1, GreaterThan14/1, GreaterThan15/1, GreaterThan18/1, GreaterThan19/1, GreaterThan12/1, GreaterThan13/1, GreaterThan10/1, GreaterThan11/1, GreaterThan9/1, GreaterThan8/1, GreaterThan6/1, GreaterThan7/1, GreaterThan4/1, GreaterThan5/1, GreaterThan2/1, GreaterThan3/1, GreaterThan/1, GreaterThan1/1
  COMM Task - Output Emulator/1(Send CAN1) -> [send_CAN1_Out_Emulator_bc1_TAG]
  COMM Task - Output Emulator/2(Receive CAN1) -> [receive_CAN1_Out_Emulator_bc1_TAG]
  COMM Task - Output Emulator/3(Send CAN2) -> [send_CAN2_Out_Emulator_bc1_TAG]
  COMM Task - Output Emulator/4(Receive CAN2) -> [receive_CAN2_Out_Emulator_bc1_TAG]

== system HANcoder_E407_TTA_Controller_v2/HANcoder STM32 Target - E407-STM32 algorithm/Global Ticks Increment/CAN Management/Matrix Cycle Manager/Subsystem/msg_count_DEBUG observer ==
  Data Store Read24 : DataStoreRead  DataStoreName=msg_count_DEBUG
  Terminator : Terminator
  wires:
  Data Store Read24/1 -> Terminator/1  "msg_count_DEBUG_s"

== system HANcoder_E407_TTA_Controller_v2/HANcoder STM32 Target - E407-STM32 algorithm/Global Ticks Increment/CAN1 Recieve/RxID_CAN/OutControl1_ID_CAN/CAN receive1 ==
  In1 : Inport
  Enabled Subsystem : Subsystem  TreatAsAtomicUnit=on
  S-Function : M-S-Function  FunctionName=sfcn_can_receive  Parameters=tsamp, canBus, outputNumber, dataType, byteOrder
  Out1 : Outport
  Out2 : Outport  Port=2
  Out3 : Outport  Port=3
  Out4 : Outport  Port=4
  Out5 : Outport  Port=5
  Out6 : Outport  Port=6
  Out7 : Outport  Port=7
  Out8 : Outport  Port=8
  Out9 : Outport  Port=9
  wires:
  S-Function/9 -> Enabled Subsystem/8(In8)
  S-Function/4 -> Enabled Subsystem/3(In3)
  S-Function/5 -> Enabled Subsystem/4(In4)
  S-Function/8 -> Enabled Subsystem/7(In7)
  S-Function/7 -> Enabled Subsystem/6(In6)
  S-Function/6 -> Enabled Subsystem/5(In5)
  Enabled Subsystem/8(Out8) -> Out9/1
  Enabled Subsystem/7(Out7) -> Out8/1
  Enabled Subsystem/6(Out6) -> Out7/1
  Enabled Subsystem/5(Out5) -> Out6/1
  Enabled Subsystem/4(Out4) -> Out5/1
  Enabled Subsystem/3(Out3) -> Out4/1
  Enabled Subsystem/2(Out2) -> Out3/1
  Enabled Subsystem/1(Out1) -> Out2/1
  S-Function/3 -> Enabled Subsystem/2(In2)
  S-Function/2 -> Enabled Subsystem/1(In1)
  S-Function/1 -> Out1/1, Enabled Subsystem/Enable
  In1/1 -> S-Function/1

== system HANcoder_E407_TTA_Controller_v2/HANcoder STM32 Target - E407-STM32 algorithm/Global Ticks Increment/CAN1 Recieve/RxID_CAN/OutControl2_ID_CAN/CAN receive1 ==
  In1 : Inport
  Enabled Subsystem : Subsystem  TreatAsAtomicUnit=on
  S-Function : M-S-Function  FunctionName=sfcn_can_receive  Parameters=tsamp, canBus, outputNumber, dataType, byteOrder
  Out1 : Outport
  Out2 : Outport  Port=2
  Out3 : Outport  Port=3
  Out4 : Outport  Port=4
  Out5 : Outport  Port=5
  Out6 : Outport  Port=6
  Out7 : Outport  Port=7
  Out8 : Outport  Port=8
  Out9 : Outport  Port=9
  wires:
  In1/1 -> S-Function/1
  S-Function/1 -> Enabled Subsystem/Enable, Out1/1
  S-Function/2 -> Enabled Subsystem/1(In1)
  S-Function/3 -> Enabled Subsystem/2(In2)
  Enabled Subsystem/1(Out1) -> Out2/1
  Enabled Subsystem/2(Out2) -> Out3/1
  Enabled Subsystem/3(Out3) -> Out4/1
  Enabled Subsystem/4(Out4) -> Out5/1
  Enabled Subsystem/5(Out5) -> Out6/1
  Enabled Subsystem/6(Out6) -> Out7/1
  Enabled Subsystem/7(Out7) -> Out8/1
  Enabled Subsystem/8(Out8) -> Out9/1
  S-Function/6 -> Enabled Subsystem/5(In5)
  S-Function/7 -> Enabled Subsystem/6(In6)
  S-Function/8 -> Enabled Subsystem/7(In7)
  S-Function/5 -> Enabled Subsystem/4(In4)
  S-Function/4 -> Enabled Subsystem/3(In3)
  S-Function/9 -> Enabled Subsystem/8(In8)

== system HANcoder_E407_TTA_Controller_v2/HANcoder STM32 Target - E407-STM32 algorithm/Global Ticks Increment/CAN1 Recieve/RxID_CAN/OutEmulator_ID_CAN/CAN receive1 ==
  In1 : Inport
  Enabled Subsystem : Subsystem  TreatAsAtomicUnit=on
  S-Function : M-S-Function  FunctionName=sfcn_can_receive  Parameters=tsamp, canBus, outputNumber, dataType, byteOrder
  Out1 : Outport
  Out2 : Outport  Port=2
  Out3 : Outport  Port=3
  Out4 : Outport  Port=4
  Out5 : Outport  Port=5
  Out6 : Outport  Port=6
  Out7 : Outport  Port=7
  Out8 : Outport  Port=8
  Out9 : Outport  Port=9
  wires:
  S-Function/9 -> Enabled Subsystem/8(In8)
  S-Function/4 -> Enabled Subsystem/3(In3)
  S-Function/5 -> Enabled Subsystem/4(In4)
  S-Function/8 -> Enabled Subsystem/7(In7)
  S-Function/7 -> Enabled Subsystem/6(In6)
  S-Function/6 -> Enabled Subsystem/5(In5)
  Enabled Subsystem/8(Out8) -> Out9/1
  Enabled Subsystem/7(Out7) -> Out8/1
  Enabled Subsystem/6(Out6) -> Out7/1
  Enabled Subsystem/5(Out5) -> Out6/1
  Enabled Subsystem/4(Out4) -> Out5/1
  Enabled Subsystem/3(Out3) -> Out4/1
  Enabled Subsystem/2(Out2) -> Out3/1
  Enabled Subsystem/1(Out1) -> Out2/1
  S-Function/3 -> Enabled Subsystem/2(In2)
  S-Function/2 -> Enabled Subsystem/1(In1)
  S-Function/1 -> Out1/1, Enabled Subsystem/Enable
  In1/1 -> S-Function/1

== system HANcoder_E407_TTA_Controller_v2/HANcoder STM32 Target - E407-STM32 algorithm/Global Ticks Increment/CAN1 Recieve/RxID_CAN/SensorValues_ID_CAN/CAN receive1 ==
  In1 : Inport
  Enabled Subsystem : Subsystem  TreatAsAtomicUnit=on
  S-Function : M-S-Function  FunctionName=sfcn_can_receive  Parameters=tsamp, canBus, outputNumber, dataType, byteOrder
  Out1 : Outport
  Out2 : Outport  Port=2
  Out3 : Outport  Port=3
  Out4 : Outport  Port=4
  Out5 : Outport  Port=5
  Out6 : Outport  Port=6
  Out7 : Outport  Port=7
  Out8 : Outport  Port=8
  Out9 : Outport  Port=9
  wires:
  In1/1 -> S-Function/1
  S-Function/1 -> Enabled Subsystem/Enable, Out1/1
  S-Function/2 -> Enabled Subsystem/1(In1)
  S-Function/3 -> Enabled Subsystem/2(In2)
  Enabled Subsystem/1(Out1) -> Out2/1
  Enabled Subsystem/2(Out2) -> Out3/1
  Enabled Subsystem/3(Out3) -> Out4/1
  Enabled Subsystem/4(Out4) -> Out5/1
  Enabled Subsystem/5(Out5) -> Out6/1
  Enabled Subsystem/6(Out6) -> Out7/1
  Enabled Subsystem/7(Out7) -> Out8/1
  Enabled Subsystem/8(Out8) -> Out9/1
  S-Function/6 -> Enabled Subsystem/5(In5)
  S-Function/7 -> Enabled Subsystem/6(In6)
  S-Function/8 -> Enabled Subsystem/7(In7)
  S-Function/5 -> Enabled Subsystem/4(In4)
  S-Function/4 -> Enabled Subsystem/3(In3)
  S-Function/9 -> Enabled Subsystem/8(In8)

== system HANcoder_E407_TTA_Controller_v2/HANcoder STM32 Target - E407-STM32 algorithm/Global Ticks Increment/CAN1 Recieve/RxID_CAN/SetValues_ID_CAN/CAN receive1 ==
  In1 : Inport
  Enabled Subsystem : Subsystem  TreatAsAtomicUnit=on
  S-Function : M-S-Function  FunctionName=sfcn_can_receive  Parameters=tsamp, canBus, outputNumber, dataType, byteOrder
  Out1 : Outport
  Out2 : Outport  Port=2
  Out3 : Outport  Port=3
  Out4 : Outport  Port=4
  Out5 : Outport  Port=5
  Out6 : Outport  Port=6
  Out7 : Outport  Port=7
  Out8 : Outport  Port=8
  Out9 : Outport  Port=9
  wires:
  S-Function/9 -> Enabled Subsystem/8(In8)
  S-Function/4 -> Enabled Subsystem/3(In3)
  S-Function/5 -> Enabled Subsystem/4(In4)
  S-Function/8 -> Enabled Subsystem/7(In7)
  S-Function/7 -> Enabled Subsystem/6(In6)
  S-Function/6 -> Enabled Subsystem/5(In5)
  Enabled Subsystem/8(Out8) -> Out9/1
  Enabled Subsystem/7(Out7) -> Out8/1
  Enabled Subsystem/6(Out6) -> Out7/1
  Enabled Subsystem/5(Out5) -> Out6/1
  Enabled Subsystem/4(Out4) -> Out5/1
  Enabled Subsystem/3(Out3) -> Out4/1
  Enabled Subsystem/2(Out2) -> Out3/1
  Enabled Subsystem/1(Out1) -> Out2/1
  S-Function/3 -> Enabled Subsystem/2(In2)
  S-Function/2 -> Enabled Subsystem/1(In1)
  S-Function/1 -> Out1/1, Enabled Subsystem/Enable
  In1/1 -> S-Function/1

== system HANcoder_E407_TTA_Controller_v2/HANcoder STM32 Target - E407-STM32 algorithm/Global Ticks Increment/CAN1 Recieve/RxID_CAN/Sync_ID_CAN/CAN receive1 ==
  In1 : Inport
  Enabled Subsystem : Subsystem  TreatAsAtomicUnit=on
  S-Function : M-S-Function  FunctionName=sfcn_can_receive  Parameters=tsamp, canBus, outputNumber, dataType, byteOrder
  Out1 : Outport
  Out2 : Outport  Port=2
  Out3 : Outport  Port=3
  Out4 : Outport  Port=4
  Out5 : Outport  Port=5
  Out6 : Outport  Port=6
  Out7 : Outport  Port=7
  Out8 : Outport  Port=8
  Out9 : Outport  Port=9
  wires:
  S-Function/9 -> Enabled Subsystem/8(In8)
  S-Function/4 -> Enabled Subsystem/3(In3)
  S-Function/5 -> Enabled Subsystem/4(In4)
  S-Function/8 -> Enabled Subsystem/7(In7)
  S-Function/7 -> Enabled Subsystem/6(In6)
  S-Function/6 -> Enabled Subsystem/5(In5)
  Enabled Subsystem/8(Out8) -> Out9/1
  Enabled Subsystem/7(Out7) -> Out8/1
  Enabled Subsystem/6(Out6) -> Out7/1
  Enabled Subsystem/5(Out5) -> Out6/1
  Enabled Subsystem/4(Out4) -> Out5/1
  Enabled Subsystem/3(Out3) -> Out4/1
  Enabled Subsystem/2(Out2) -> Out3/1
  Enabled Subsystem/1(Out1) -> Out2/1
  S-Function/3 -> Enabled Subsystem/2(In2)
  S-Function/2 -> Enabled Subsystem/1(In1)
  S-Function/1 -> Out1/1, Enabled Subsystem/Enable
  In1/1 -> S-Function/1
